simulink library "TM_DynamicModel_Library"  (Simulink 7.8)
settings: Solver=ode45  StartTime=0.0  StopTime=10.0  RelTol=1e-3
undefined symbols (not defined in the file or in its folder): DiscIntNeverNeededParam
libraries: simulink x43, TM_DynamicModel_Library x7
(part 1 of 2)
settings Model: Creator=vpadmaj  LastModifiedBy=vpadmaj

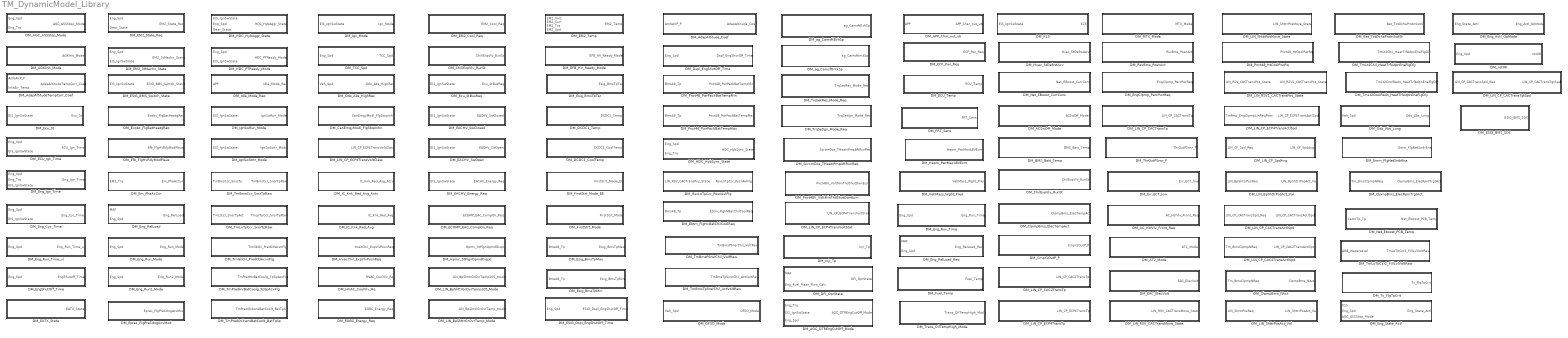
== system TM_DynamicModel_Library ==
  DM_ACSwOff_Mode : Subsystem
  DM_AC_HtrVlv_Front_Req : Subsystem
  DM_AGC_ASSStop_Mode : Subsystem
  DM_AGC_DTREngCutOff_Mode : Subsystem
  DM_AGKInit_Mode : Subsystem
  DM_APP_Char_out_ub : Subsystem
  DM_AT2_Mode : Subsystem
  DM_AdapAltitudeTempCorr_Coef : Subsystem
  DM_AdapAltitude_Coef : Subsystem
  DM_BMS_Batt_Temp : Subsystem
  DM_Bat_TotDchaProtnSwtSt : Subsystem
  DM_CanEmgyModl_FlgStopInhn : Subsystem
  DM_ChilExpVlv_RunSt : Subsystem
  DM_ChillExpVlv_RunSt : Subsystem
  DM_ClpmpBms_ElecRpmTrgtAct : Subsystem
  DM_ClpmpBms_ElecTempAct : Subsystem
  DM_ClpmpBms_NAct : Subsystem
  DM_Cmpr1OutP_P : Subsystem
  DM_DCDC1_CoolTemp : Subsystem
  DM_DCDC1_Temp : Subsystem
  DM_DFI_OprState : Subsystem
  DM_DFSO_Mode : Subsystem
  DM_Dspl_EngShutOff_Time : Subsystem
  DM_EACHV_Energy_Req : Subsystem
  DM_EACHV_SwClosed : Subsystem
  DM_EACHV_SwOpen : Subsystem
  DM_EAC_ElecVolt : Subsystem
  DM_EATX_State : Subsystem
  DM_ECF_Pwr_Req : Subsystem
  DM_ECOMP_EAC_CompOn_Req : Subsystem
  DM_ECU_Ign_Time : Subsystem
  DM_ECU_Temp : Subsystem
  DM_EFB_HV_Ready_Mode : Subsystem
  DM_EM2_Cool_Req : Subsystem
  DM_EM2_StMachn_State : Subsystem
  DM_EM2_State_Req : Subsystem
  DM_EM2_Temp : Subsystem
  DM_EOBC_Energy_Req : Subsystem
  DM_ESIG_BMS_SOC : Subsystem
  DM_ESIG_BMS_Switch_State : Subsystem
  DM_ESIG_Dspl_EngShutOff_Time : Subsystem
  DM_Ebtm_FlgHvBatChilCoolReq : Subsystem
  DM_Ecobc_FlgBatHeatgReq : Subsystem
  DM_Ecu_St : Subsystem
  DM_Ecu_StBusReq : Subsystem
  DM_Efb_FlgHvRdyModPlaus : Subsystem
  DM_Em_PhaAcCur : Subsystem
  DM_Emm_FlgNetSndrEna : Subsystem
  DM_EngClpmp_PercPwrReq : Subsystem
  DM_EngShutOff_Time : Subsystem
  DM_Eng_Actl_OpMode : Subsystem
  DM_Eng_Cyc_Time : Subsystem
  DM_Eng_Ign_Time : Subsystem
  DM_Eng_RelLoad : Subsystem
  DM_Eng_RelLoad_Req : Subsystem
  DM_Eng_Run2_Mode : Subsystem
  DM_Eng_Run_Mode : Subsystem
  DM_Eng_Run_Time : Subsystem
  DM_Eng_Run_Time_ul : Subsystem
  DM_Eng_State_Actl : Subsystem
  DM_Eprec_FlgPreCdngAcvMod : Subsystem
  DM_Err_ECT_low : Subsystem
  DM_Esig_BmsTpMax : Subsystem
  DM_Esig_BmsTpMin : Subsystem
  DM_Esig_BmsTpTar : Subsystem
  DM_FRT_Sens : Subsystem
  DM_FirstStrt_Mode : Subsystem
  DM_FirstStrt_Mode_EE : Subsystem
  DM_Fuel_Temp : Subsystem
  DM_HDC_HybAggr_State : Subsystem
  DM_HDC_HybSync_State : Subsystem
  DM_HDC_PTReady_Mode : Subsystem
  DM_HVAC_CoolVlv_Rq : Subsystem
  DM_Hepm_PwrMax48VEcm : Subsystem
  DM_Hpmc_StPlgnOpmdDispd : Subsystem
  DM_HvacChil_ExpVlvPosnReq : Subsystem
  DM_Hvac_StDefrstAcv : Subsystem
  DM_IC_Knk_Red_Avg : Subsystem
  DM_IC_Knk_Red_Avg_Actv : Subsystem
  DM_Idle_Mode_Req : Subsystem
  DM_IgnSwRun_Mode : Subsystem
  DM_IgnSwStrtr_Mode : Subsystem
  DM_Ign_Mode : Subsystem
  DM_Injr_Tp : Subsystem
  DM_K15 : Subsystem
  DM_LIN_BpShttrGrOvrTemp105_Mode : Subsystem
  DM_LIN_BpShttrGrOvrTemp_Mode : Subsystem
  DM_LIN_BpShttrPosAct_Val : Subsystem
  DM_LIN_CF_SpdAvg : Subsystem
  DM_LIN_CP_CAC2TransActlSpd : Subsystem
  DM_LIN_CP_CAC2TransTp : Subsystem
  DM_LIN_CP_CACTransActlSpd : Subsystem
  DM_LIN_CP_CACTransTgtSpd : Subsystem
  DM_LIN_CP_CACTransTp : Subsystem
  DM_LIN_CP_ECP4TransActlSpd : Subsystem
  DM_LIN_CP_ECP4TransTp : Subsystem
  DM_LIN_CP_ECP4TransVoltClass : Subsystem
  DM_LIN_CP_ECP4TransVoltStat : Subsystem
  DM_LIN_RSV1_CACTransPos_State : Subsystem
  DM_LIN_RSV_CACTransMove_State : Subsystem
  DM_LIN_ShttrPosAct_Val : Subsystem
  DM_LIN_ShttrPosMove_State : Subsystem
  DM_MTX_Mode : Subsystem
  DM_Net_EBoost_CurrCons : Subsystem
  DM_Net_Eboost_PCB_Temp : Subsystem
  DM_Odo_Abs_HighRes : Subsystem
  DM_Odo_Abs_Long : Subsystem
  DM_Pnct48V_VoltMinThdShutDwnEcm : Subsystem
  DM_Pnct48_HtCoolPwrRq : Subsystem
  DM_Pnct48_PwrPackBatTempMax : Subsystem
  DM_Pnct48_PwrPackBatTempMin : Subsystem
  DM_RsvBms_PosnAct : Subsystem
  DM_RsvLoTpCcr_PosnAvlFlg : Subsystem
  DM_ScrcmDos_THeatrPmpAftRunReq : Subsystem
  DM_TCC_Spd : Subsystem
  DM_Tc_FlgTpCrit : Subsystem
  DM_ThrOutPSnsr_P : Subsystem
  DM_TmBmsCcr_SnsrTpRaw : Subsystem
  DM_TmBmsPSnsrChil_VoltRaw : Subsystem
  DM_TmBmsTpSnsrChil_ActVoltRaw : Subsystem
  DM_TmGbOil_PredCtlAcvnFlg : Subsystem
  DM_TmLoTpCcr2_FillLvlVoltRaw : Subsystem
  DM_TmLoTpCcr_SnsrTpRaw : Subsystem
  DM_TmLt2Chil_HeatTrfAdpnEnaFlgDly : Subsystem
  DM_TmLt2CoolRedn_HeatTrfAdpnEnaFlgDly : Subsystem
  DM_TmPredHvBatCoolg_TpSpAcvFlg : Subsystem
  DM_TmPredQckwnsBatCoolt_BatTpSp : Subsystem
  DM_Trans_OilTempHigh_Mode : Subsystem
  DM_TrqSetIgn_Mode_Req : Subsystem
  DM_TrqSetRes_Mode_Req : Subsystem
  DM_VehMass_Wght_Pred : Subsystem
  DM_ag_CamsftExhSp : Subsystem
  DM_ag_CamsftIntkSp : Subsystem
  DM_nst08 : Subsystem

== system TM_DynamicModel_Library/DM_ACSwOff_Mode ==
  Constant : Constant
  ACSwOff_Mode : Outport
  wires:
  Constant/1 -> ACSwOff_Mode/1

== system TM_DynamicModel_Library/DM_AC_HtrVlv_Front_Req ==
  Constant : Constant
  AC_HtrVlv_Front_Req : Outport
  wires:
  Constant/1 -> AC_HtrVlv_Front_Req/1

== system TM_DynamicModel_Library/DM_AGC_ASSStop_Mode ==
  Eng_Spd : Inport
  Eng_Trq : Inport  Port=2
  Add : Sum  Inputs=+-
  Constant : Constant  Value=0
  Constant1 : Constant  Value=-100
  Constant2 : Constant  Value=0
  Data Type Conversion : DataTypeConversion
  Logical Operator : Logic  AllPortsSameDT=off  OutDataTypeStr=boolean
  Logical Operator1 : Logic  Operator=NOR  AllPortsSameDT=off  OutDataTypeStr=boolean
  Relational Operator : RelationalOperator  Operator=>  OutDataTypeStr=boolean
  Relational Operator1 : RelationalOperator  Operator=<  OutDataTypeStr=boolean
  Relational Operator2 : RelationalOperator  Operator=>  OutDataTypeStr=boolean
  Unit Delay : UnitDelay  SampleTime=-1
  AGC_ASSStop_Mode : Outport
  wires:
  Data Type Conversion/1 -> AGC_ASSStop_Mode/1
  Constant/1 -> Relational Operator/2
  Eng_Spd/1 -> Relational Operator/1, Unit Delay/1, Add/1
  Relational Operator/1 -> Logical Operator1/1
  Unit Delay/1 -> Add/2
  Constant1/1 -> Relational Operator1/2
  Add/1 -> Relational Operator1/1
  Constant2/1 -> Relational Operator2/2
  Eng_Trq/1 -> Relational Operator2/1
  Relational Operator1/1 -> Logical Operator/1
  Relational Operator2/1 -> Logical Operator/2
  Logical Operator/1 -> Logical Operator1/2
  Logical Operator1/1 -> Data Type Conversion/1

== system TM_DynamicModel_Library/DM_AGC_DTREngCutOff_Mode ==
  Eng_Trq : Inport
  EIS_IgnSwState : Inport  Port=2
  Eng_Spd : Inport  Port=3
  Constant3 : Constant  Value=0
  DM_AGC_ASSStop_Mode : TM_DynamicModel_Library/DM_AGC_ASSStop_Mode
  DM_Ign_Mode : Subsystem
  Data Type Conversion : DataTypeConversion
  Logical Operator1 : Logic  AllPortsSameDT=off  OutDataTypeStr=boolean
  Logical Operator2 : Logic  Operator=OR  AllPortsSameDT=off  OutDataTypeStr=boolean
  Relational Operator4 : RelationalOperator  Operator=<=  OutDataTypeStr=boolean
  AGC_DTREngCutOff_Mode : Outport
  wires:
  Data Type Conversion/1 -> AGC_DTREngCutOff_Mode/1
  Constant3/1 -> Relational Operator4/2
  Eng_Spd/1 -> Relational Operator4/1, DM_AGC_ASSStop_Mode/1
  Relational Operator4/1 -> Logical Operator1/2
  Logical Operator1/1 -> Logical Operator2/2
  Logical Operator2/1 -> Data Type Conversion/1
  DM_AGC_ASSStop_Mode/1 -> Logical Operator2/1
  EIS_IgnSwState/1 -> DM_Ign_Mode/1(EIS_IgnSwState)
  Eng_Trq/1 -> DM_AGC_ASSStop_Mode/2
  DM_Ign_Mode/1(Ign_Mode) -> Logical Operator1/1

== system TM_DynamicModel_Library/DM_AGKInit_Mode ==
  note: This variable is a part of DC_SP function. Current implementation is from page 1210
      | of function definition document for M256 16A_Star23_VC05 L03FRG
  0 : UnitDelay  SampleTime=-1
  1 : UnitDelay  X0=1  SampleTime=-1
  Add : Sum
  Constant : Constant
  Constant1 : Constant  Value=0
  Data Type Conversion : DataTypeConversion
  Logical Operator : Logic  Operator=NOT  AllPortsSameDT=off  OutDataTypeStr=boolean
  Logical Operator1 : Logic  AllPortsSameDT=off  OutDataTypeStr=boolean
  Relational Operator : RelationalOperator  Operator===  OutDataTypeStr=boolean
  Switch : Switch  Threshold=1
  "This constant value has been changed from 10 to 1, because this function is now being called every 0.1s instead of 0.01s" : Constant  Value=10
  AGKInit_Mode : Outport
  wires:
  Data Type Conversion/1 -> AGKInit_Mode/1
  Switch/1 -> Add/2
  Add/1 -> 0/1
  "This constant value has been changed from 10 to 1, because this function is now being called every 0.1s instead of 0.01s"/1 -> Relational Operator/2
  0/1 -> Relational Operator/1, Add/1
  Relational Operator/1 -> Logical Operator/1, Switch/2
  Logical Operator/1 -> Logical Operator1/1
  1/1 -> Logical Operator1/2
  Logical Operator1/1 -> Data Type Conversion/1, 1/1
  Constant1/1 -> Switch/1
  Constant/1 -> Switch/3

== system TM_DynamicModel_Library/DM_APP_Char_out_ub ==
  APP : Inport
  Characterisation : Lookup  InputValues=[0,10,20,30,40,50,60,70,80,90,100]  Table=[0,8,17,26,35,44,59,70,82,91,100]
  APP_Char_out_ub : Outport
  wires:
  APP/1 -> Characterisation/1
  Characterisation/1 -> APP_Char_out_ub/1

== system TM_DynamicModel_Library/DM_AT2_Mode ==
  Constant : Constant  Value=0
  AT2_Mode : Outport
  wires:
  Constant/1 -> AT2_Mode/1

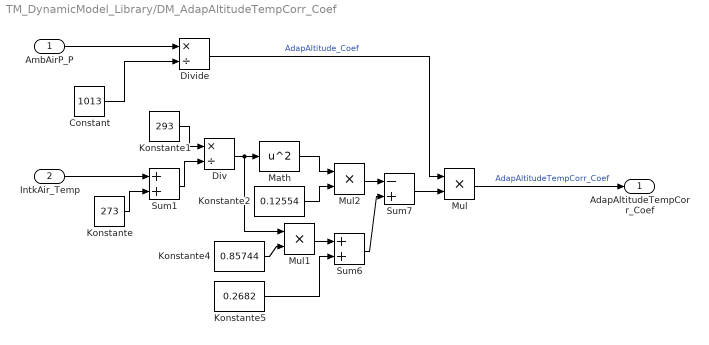
== system TM_DynamicModel_Library/DM_AdapAltitudeTempCorr_Coef ==
  AmbAirP_P : Inport
  IntkAir_Temp : Inport  Port=2  PortDimensions=1
  Constant : Constant  Value=1013
  Div : Product  Tag=COPIED_DURING_UPGRADE  Description=|  Inputs=*/  RndMeth=Zero  mask(TL_Product){data={'logdata',{'plotchannels',[]},'output',{'type','DC_FCTR_32768_U16'},'date',734244.44671856484}}
      | Product block of dSPACE TargetLink.
      | 
      | Output signal is equal to the product of the input signals. The input ports are specified according to conventions for Simulink Product blocks.
      settings: DeleteFcn=if exist('delete_tlblock','file')==2,delete_tlblock(gcbh);end  NameChangeFcn=if exist('rename_tlblock','file')==2,rename_tlblock(gcbh);end  OpenFcn=if exist('tl_open_blockdlg','file')==2,tl_open_blockdlg(gcbh);else,open_system(gcbh,'parameter');end
      mask Help: eval(['if exist(''tl_online_help'',''file'') == 2, tl_online_help(''Topic'',''TL_Product''),else, web([''jar:file:///'',matlabroot,''/help/toolbox/simulink/help.jar!/slref/' lower(get_param(gcbh,'Blocktype')) '.html''], ''-helpbrowser''),end'])
  Divide : Product  Inputs=*/
  Konstante : Constant  Tag=COPIED_DURING_UPGRADE  Description=|  Value=273
      | Constant block of dSPACE TargetLink.
      | 
      | Output signal keeps the given constant value.
      settings: DeleteFcn=if exist('delete_tlblock','file')==2,delete_tlblock(gcbh);end  NameChangeFcn=if exist('rename_tlblock','file')==2,rename_tlblock(gcbh);end  OpenFcn=if exist('tl_open_blockdlg','file')==2,tl_open_blockdlg(gcbh);else,open_system(gcbh,'parameter');end
  Konstante1 : Constant  Tag=COPIED_DURING_UPGRADE  Description=|  Value=293  mask(TL_Constant){data={'date',734244.44671675924}}
      | Constant block of dSPACE TargetLink.
      | 
      | Output signal keeps the given constant value.
      settings: DeleteFcn=if exist('delete_tlblock','file')==2,delete_tlblock(gcbh);end  NameChangeFcn=if exist('rename_tlblock','file')==2,rename_tlblock(gcbh);end  OpenFcn=if exist('tl_open_blockdlg','file')==2,tl_open_blockdlg(gcbh);else,open_system(gcbh,'parameter');end
      mask Help: eval(['if exist(''tl_online_help'',''file'') == 2, tl_online_help(''Topic'',''TL_Constant''),else, web([''jar:file:///'',matlabroot,''/help/toolbox/simulink/help.jar!/slref/' lower(get_param(gcbh,'Blocktype')) '.html''], ''-helpbrowser''),end'])
  Konstante2 : Constant  Tag=COPIED_DURING_UPGRADE  Description=|  Value=0.12554
      | Constant block of dSPACE TargetLink.
      | 
      | Output signal keeps the given constant value.
      settings: DeleteFcn=if exist('delete_tlblock','file')==2,delete_tlblock(gcbh);end  NameChangeFcn=if exist('rename_tlblock','file')==2,rename_tlblock(gcbh);end  OpenFcn=if exist('tl_open_blockdlg','file')==2,tl_open_blockdlg(gcbh);else,open_system(gcbh,'parameter');end
  Konstante4 : Constant  Tag=COPIED_DURING_UPGRADE  Description=|  Value=0.85744
      | Constant block of dSPACE TargetLink.
      | 
      | Output signal keeps the given constant value.
      settings: DeleteFcn=if exist('delete_tlblock','file')==2,delete_tlblock(gcbh);end  NameChangeFcn=if exist('rename_tlblock','file')==2,rename_tlblock(gcbh);end  OpenFcn=if exist('tl_open_blockdlg','file')==2,tl_open_blockdlg(gcbh);else,open_system(gcbh,'parameter');end
  Konstante5 : Constant  Tag=COPIED_DURING_UPGRADE  Description=|  Value=0.2682
      | Constant block of dSPACE TargetLink.
      | 
      | Output signal keeps the given constant value.
      settings: DeleteFcn=if exist('delete_tlblock','file')==2,delete_tlblock(gcbh);end  NameChangeFcn=if exist('rename_tlblock','file')==2,rename_tlblock(gcbh);end  OpenFcn=if exist('tl_open_blockdlg','file')==2,tl_open_blockdlg(gcbh);else,open_system(gcbh,'parameter');end
  Math : Math  Tag=COPIED_DURING_UPGRADE  Description=|  Operator=square  SaturateOnIntegerOverflow=on
      | Math block of dSPACE TargetLink.
      | 
      | The Math block outputs the result of the specified math function applied to the input(s). Note that unlike Simulink's Math block, this block does not support complex signals.
      settings: DeleteFcn=if exist('delete_tlblock','file')==2,delete_tlblock(gcbh);end  NameChangeFcn=if exist('rename_tlblock','file')==2,rename_tlblock(gcbh);end  OpenFcn=if exist('tl_open_blockdlg','file')==2,tl_open_blockdlg(gcbh);else,open_system(gcbh,'parameter');end
  Mul : Product  Tag=COPIED_DURING_UPGRADE  Description=|  RndMeth=Zero
      | Product block of dSPACE TargetLink.
      | 
      | Output signal is equal to the product of the input signals. The input ports are specified according to conventions for Simulink Product blocks.
      settings: DeleteFcn=if exist('delete_tlblock','file')==2,delete_tlblock(gcbh);end  NameChangeFcn=if exist('rename_tlblock','file')==2,rename_tlblock(gcbh);end  OpenFcn=if exist('tl_open_blockdlg','file')==2,tl_open_blockdlg(gcbh);else,open_system(gcbh,'parameter');end
  Mul1 : Product  Tag=COPIED_DURING_UPGRADE  Description=|  RndMeth=Zero
      | Product block of dSPACE TargetLink.
      | 
      | Output signal is equal to the product of the input signals. The input ports are specified according to conventions for Simulink Product blocks.
      settings: DeleteFcn=if exist('delete_tlblock','file')==2,delete_tlblock(gcbh);end  NameChangeFcn=if exist('rename_tlblock','file')==2,rename_tlblock(gcbh);end  OpenFcn=if exist('tl_open_blockdlg','file')==2,tl_open_blockdlg(gcbh);else,open_system(gcbh,'parameter');end
  Mul2 : Product  Tag=COPIED_DURING_UPGRADE  Description=|  RndMeth=Zero
      | Product block of dSPACE TargetLink.
      | 
      | Output signal is equal to the product of the input signals. The input ports are specified according to conventions for Simulink Product blocks.
      settings: DeleteFcn=if exist('delete_tlblock','file')==2,delete_tlblock(gcbh);end  NameChangeFcn=if exist('rename_tlblock','file')==2,rename_tlblock(gcbh);end  OpenFcn=if exist('tl_open_blockdlg','file')==2,tl_open_blockdlg(gcbh);else,open_system(gcbh,'parameter');end
  Sum1 : Sum  Tag=COPIED_DURING_UPGRADE  Description=|
      | Sum block of dSPACE TargetLink.
      | 
      | Output signal is equal to the sum of the input signals.
      | The list of signs is specified according to conventions for Simulink Sum blocks.
      settings: DeleteFcn=if exist('delete_tlblock','file')==2,delete_tlblock(gcbh);end  NameChangeFcn=if exist('rename_tlblock','file')==2,rename_tlblock(gcbh);end  OpenFcn=if exist('tl_open_blockdlg','file')==2,tl_open_blockdlg(gcbh);else,open_system(gcbh,'parameter');end
  Sum6 : Sum  Tag=COPIED_DURING_UPGRADE  Description=|
      | Sum block of dSPACE TargetLink.
      | 
      | Output signal is equal to the sum of the input signals.
      | The list of signs is specified according to conventions for Simulink Sum blocks.
      settings: DeleteFcn=if exist('delete_tlblock','file')==2,delete_tlblock(gcbh);end  NameChangeFcn=if exist('rename_tlblock','file')==2,rename_tlblock(gcbh);end  OpenFcn=if exist('tl_open_blockdlg','file')==2,tl_open_blockdlg(gcbh);else,open_system(gcbh,'parameter');end
  Sum7 : Sum  Tag=COPIED_DURING_UPGRADE  Description=|  Inputs=-+
      | Sum block of dSPACE TargetLink.
      | 
      | Output signal is equal to the sum of the input signals.
      | The list of signs is specified according to conventions for Simulink Sum blocks.
      settings: DeleteFcn=if exist('delete_tlblock','file')==2,delete_tlblock(gcbh);end  NameChangeFcn=if exist('rename_tlblock','file')==2,rename_tlblock(gcbh);end  OpenFcn=if exist('tl_open_blockdlg','file')==2,tl_open_blockdlg(gcbh);else,open_system(gcbh,'parameter');end
  AdapAltitudeTempCorr_Coef : Outport
  wires:
  AmbAirP_P/1 -> Divide/1
  IntkAir_Temp/1 -> Sum1/1
  Mul/1 -> AdapAltitudeTempCorr_Coef/1  "AdapAltitudeTempCorr_Coef"
  Constant/1 -> Divide/2
  Sum7/1 -> Mul/2
  Mul2/1 -> Sum7/1
  Sum6/1 -> Sum7/2
  Math/1 -> Mul2/1
  Div/1 -> Mul1/1, Math/1
  Konstante2/1 -> Mul2/2
  Konstante4/1 -> Mul1/2
  Mul1/1 -> Sum6/1
  Konstante5/1 -> Sum6/2
  Konstante1/1 -> Div/1
  Sum1/1 -> Div/2
  Konstante/1 -> Sum1/2
  Divide/1 -> Mul/1  "AdapAltitude_Coef"

== system TM_DynamicModel_Library/DM_AdapAltitude_Coef ==
  AmbAirP_P : Inport
  Constant : Constant  Value=1013
  Divide : Product  Inputs=*/
  AdapAltitude_Coef : Outport
  wires:
  AmbAirP_P/1 -> Divide/1
  Constant/1 -> Divide/2
  Divide/1 -> AdapAltitude_Coef/1  "AdapAltitude_Coef"

== system TM_DynamicModel_Library/DM_BMS_Batt_Temp ==
  Constant : Constant  Value=30
  BMS_Batt_Temp : Outport
  wires:
  Constant/1 -> BMS_Batt_Temp/1

== system TM_DynamicModel_Library/DM_Bat_TotDchaProtnSwtSt ==
  Constant : Constant
  Bat_TotDchaProtnSwtSt : Outport
  wires:
  Constant/1 -> Bat_TotDchaProtnSwtSt/1

== system TM_DynamicModel_Library/DM_CanEmgyModl_FlgStopInhn ==
  Constant : Constant  Value=0
  CanEmgyModl_FlgStopInhn : Outport
  wires:
  Constant/1 -> CanEmgyModl_FlgStopInhn/1

== system TM_DynamicModel_Library/DM_ChilExpVlv_RunSt ==
  Constant : Constant  Value=0
  ChilExpVlv_RunSt : Outport
  wires:
  Constant/1 -> ChilExpVlv_RunSt/1

== system TM_DynamicModel_Library/DM_ChillExpVlv_RunSt ==
  Constant : Constant  Value=0
  ChillExpVlv_RunSt : Outport
  wires:
  Constant/1 -> ChillExpVlv_RunSt/1

== system TM_DynamicModel_Library/DM_ClpmpBms_ElecRpmTrgtAct ==
  Tm_BmsClpmpNReq : Inport
  Unit Delay : UnitDelay  SampleTime=-1
  ClpmpBms_ElecRpmTrgtAct : Outport
  wires:
  Unit Delay/1 -> ClpmpBms_ElecRpmTrgtAct/1
  Tm_BmsClpmpNReq/1 -> Unit Delay/1

== system TM_DynamicModel_Library/DM_ClpmpBms_ElecTempAct ==
  Constant : Constant  Value=40
  ClpmpBms_ElecTempAct : Outport
  wires:
  Constant/1 -> ClpmpBms_ElecTempAct/1

== system TM_DynamicModel_Library/DM_ClpmpBms_NAct ==
  Tm_BmsClpmpNReq : Inport
  Unit Delay : UnitDelay  SampleTime=-1
  Unit Delay1 : UnitDelay  SampleTime=-1
  ClpmpBms_NAct : Outport
  wires:
  Tm_BmsClpmpNReq/1 -> Unit Delay/1
  Unit Delay/1 -> Unit Delay1/1
  Unit Delay1/1 -> ClpmpBms_NAct/1

== system TM_DynamicModel_Library/DM_Cmpr1OutP_P ==
  Constant : Constant  Value=1000
  Cmpr1OutP_P : Outport
  wires:
  Constant/1 -> Cmpr1OutP_P/1

== system TM_DynamicModel_Library/DM_DCDC1_CoolTemp ==
  Constant : Constant  Value=30
  DCDC1_CoolTemp : Outport
  wires:
  Constant/1 -> DCDC1_CoolTemp/1

== system TM_DynamicModel_Library/DM_DCDC1_Temp ==
  Constant : Constant  Value=30
  DCDC1_Temp : Outport
  wires:
  Constant/1 -> DCDC1_Temp/1

== system TM_DynamicModel_Library/DM_DFI_OprState ==
  MAF : Inport
  Eng_Fuel_Mass_Flow_Calc : Inport  Port=2
  Constant : Constant  Value=65
  Constant1 : Constant
  Constant2 : Constant  Value=1.06
  Divide : Product  Inputs=*/
  Relational Operator : RelationalOperator  Operator=<  OutDataTypeStr=boolean
  Saturation : Saturate  UpperLimit=inf  LowerLimit=eps
  Switch : Switch
  kgph_2_gpmin : Gain  Gain=60/1000
  DFI_OprState : Outport
  wires:
  kgph_2_gpmin/1 -> Divide/1
  MAF/1 -> kgph_2_gpmin/1
  Eng_Fuel_Mass_Flow_Calc/1 -> Saturation/1
  Divide/1 -> Relational Operator/1
  Relational Operator/1 -> Switch/2
  Switch/1 -> DFI_OprState/1
  Constant/1 -> Switch/1
  Constant1/1 -> Switch/3
  Constant2/1 -> Relational Operator/2
  Saturation/1 -> Divide/2

== system TM_DynamicModel_Library/DM_DFSO_Mode ==
  Veh_Spd : Inport
  Constant1 : Constant  Value=-0.7
  Data Type Conversion : DataTypeConversion
  Derivative : Derivative
  Gain2 : Gain  Gain=0.4
  Relational Operator : RelationalOperator  OutDataTypeStr=boolean
  DFSO_Mode : Outport
  wires:
  Data Type Conversion/1 -> DFSO_Mode/1
  Derivative/1 -> Gain2/1
  Gain2/1 -> Relational Operator/2
  Constant1/1 -> Relational Operator/1
  Relational Operator/1 -> Data Type Conversion/1
  Veh_Spd/1 -> Derivative/1

== system TM_DynamicModel_Library/DM_Dspl_EngShutOff_Time ==
  Eng_Spd : Inport
  DM_EngShutoff_Time : Subsystem
  Dspl_EngShutOff_Time : Outport
  wires:
  Eng_Spd/1 -> DM_EngShutoff_Time/1(Eng_Spd)
  DM_EngShutoff_Time/1(EngShutoff_Time) -> Dspl_EngShutOff_Time/1

== system TM_DynamicModel_Library/DM_EACHV_Energy_Req ==
  EIS_IgnSwState : Inport
  Constant : Constant  Value=4
  DM_Ecu_St : Subsystem
  Data Type Conversion : DataTypeConversion
  Relational Operator : RelationalOperator  Operator===  OutDataTypeStr=boolean
  EACHV_Energy_Req : Outport
  wires:
  Data Type Conversion/1 -> EACHV_Energy_Req/1
  Constant/1 -> Relational Operator/2
  Relational Operator/1 -> Data Type Conversion/1
  EIS_IgnSwState/1 -> DM_Ecu_St/1(EIS_IgnSwState)
  DM_Ecu_St/1(Ecu_St) -> Relational Operator/1

== system TM_DynamicModel_Library/DM_EACHV_SwClosed ==
  EIS_IgnSwState : Inport
  Constant : Constant  Value=2
  DM_ESIG_BMS_Switch_State : Subsystem
  Data Type Conversion : DataTypeConversion
  Relational Operator : RelationalOperator  Operator===  OutDataTypeStr=boolean
  EACHV_SwClosed : Outport
  wires:
  Data Type Conversion/1 -> EACHV_SwClosed/1
  Constant/1 -> Relational Operator/2
  Relational Operator/1 -> Data Type Conversion/1
  EIS_IgnSwState/1 -> DM_ESIG_BMS_Switch_State/1(EIS_IgnSwState)
  DM_ESIG_BMS_Switch_State/1(ESIG_BMS_Switch_State) -> Relational Operator/1

== system TM_DynamicModel_Library/DM_EACHV_SwOpen ==
  EIS_IgnSwState : Inport
  Constant : Constant  Value=2
  DM_ESIG_BMS_Switch_State : Subsystem
  Data Type Conversion : DataTypeConversion
  Logical Operator : Logic  Operator=NOT  AllPortsSameDT=off  OutDataTypeStr=boolean
  Relational Operator : RelationalOperator  Operator===  OutDataTypeStr=boolean
  EACHV_SwOpen : Outport
  wires:
  Data Type Conversion/1 -> EACHV_SwOpen/1
  Constant/1 -> Relational Operator/2
  Relational Operator/1 -> Logical Operator/1
  Logical Operator/1 -> Data Type Conversion/1
  EIS_IgnSwState/1 -> DM_ESIG_BMS_Switch_State/1(EIS_IgnSwState)
  DM_ESIG_BMS_Switch_State/1(ESIG_BMS_Switch_State) -> Relational Operator/1

== system TM_DynamicModel_Library/DM_EAC_ElecVolt ==
  Constant : Constant  Value=48
  EAC_ElecVolt : Outport
  wires:
  Constant/1 -> EAC_ElecVolt/1

== system TM_DynamicModel_Library/DM_EATX_State ==
  Constant : Constant  Value=4
  EATX_State : Outport
  wires:
  Constant/1 -> EATX_State/1

== system TM_DynamicModel_Library/DM_ECF_Pwr_Req ==
  Constant : Constant  Value=0
  ECF_Pwr_Req : Outport
  wires:
  Constant/1 -> ECF_Pwr_Req/1

== system TM_DynamicModel_Library/DM_ECOMP_EAC_CompOn_Req ==
  Constant : Constant  Value=0
  ECOMP_EAC_CompOn_Req : Outport
  wires:
  Constant/1 -> ECOMP_EAC_CompOn_Req/1

== system TM_DynamicModel_Library/DM_ECU_Ign_Time ==
  Eng_Spd : Inport
  EIS_IgnSwState : Inport  Port=2
  Constant46 : Constant  Value=0
  Constant47 : Constant  Value=0
  Constant48 : Constant  Value=0
  Counter_RE : Subsystem
  EdgeBi : Subsystem
  Eng_Run2_Mode_Sys : TM_DynamicModel_Library/DM_Eng_Run2_Mode
  Gain : Gain  Gain=0.01
  IgnSwRun_Mode : Subsystem
  Unit Delay3 : UnitDelay  SampleTime=-1
  ECU_Ign_Time : Outport
  wires:
  Constant46/1 -> Counter_RE/3(InitVal)
  EdgeBi/1(y) -> Counter_RE/2(Reset)
  Unit Delay3/1 -> EdgeBi/2(R)
  Constant47/1 -> EdgeBi/3(IV)
  Constant48/1 -> Unit Delay3/1
  Eng_Run2_Mode_Sys/1 -> Counter_RE/1(Enable)
  Counter_RE/1(y) -> Gain/1
  Gain/1 -> ECU_Ign_Time/1
  Eng_Spd/1 -> Eng_Run2_Mode_Sys/1
  IgnSwRun_Mode/1(IgnSwRun_Mode) -> EdgeBi/1(u)
  EIS_IgnSwState/1 -> IgnSwRun_Mode/1(IgnKeyPosition)

== system TM_DynamicModel_Library/DM_ECU_Temp ==
  Constant : Constant  Value=30
  ECU_Temp : Outport
  wires:
  Constant/1 -> ECU_Temp/1

== system TM_DynamicModel_Library/DM_EFB_HV_Ready_Mode ==
  Constant : Constant
  EFB_HV_Ready_Mode : Outport
  wires:
  Constant/1 -> EFB_HV_Ready_Mode/1

== system TM_DynamicModel_Library/DM_EM2_Cool_Req ==
  Constant : Constant  Value=0
  EM2_Cool_Req : Outport
  wires:
  Constant/1 -> EM2_Cool_Req/1

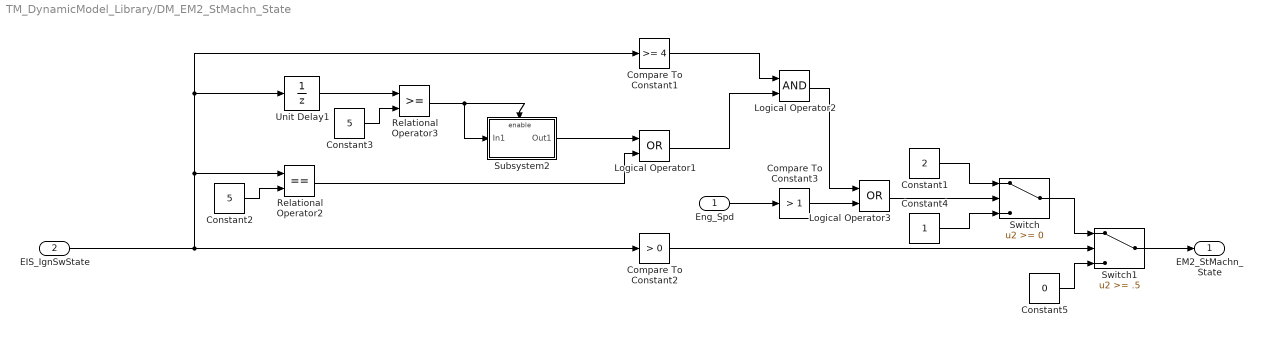
== system TM_DynamicModel_Library/DM_EM2_StMachn_State ==
  Eng_Spd : Inport
  EIS_IgnSwState : Inport  Port=2
  Compare To Constant1 : simulink/Logic and Bit Operations/Compare To Constant  relop=>=  const=4  OutDataTypeStr=uint8
  Compare To Constant2 : simulink/Logic and Bit Operations/Compare To Constant  relop=>  const=0  OutDataTypeStr=uint8
  Compare To Constant3 : simulink/Logic and Bit Operations/Compare To Constant  relop=>  const=1  OutDataTypeStr=uint8
  Constant1 : Constant  Value=2
  Constant2 : Constant  Value=5
  Constant3 : Constant  Value=5
  Constant4 : Constant
  Constant5 : Constant  Value=0
  Logical Operator1 : Logic  Operator=OR  AllPortsSameDT=off  OutDataTypeStr=boolean
  Logical Operator2 : Logic  AllPortsSameDT=off  OutDataTypeStr=boolean
  Logical Operator3 : Logic  Operator=OR  AllPortsSameDT=off  OutDataTypeStr=boolean
  Relational Operator2 : RelationalOperator  Operator===  OutDataTypeStr=boolean
  Relational Operator3 : RelationalOperator  OutDataTypeStr=boolean
  Subsystem2 : Subsystem
  Switch : Switch
  Switch1 : Switch  Threshold=.5
  Unit Delay1 : UnitDelay  SampleTime=-1
  EM2_StMachn_State : Outport
  wires:
  EIS_IgnSwState/1 -> Relational Operator2/1, Compare To Constant1/1, Unit Delay1/1, Compare To Constant2/1
  Constant2/1 -> Relational Operator2/2
  Unit Delay1/1 -> Relational Operator3/1
  Constant3/1 -> Relational Operator3/2
  Relational Operator2/1 -> Logical Operator1/2
  Subsystem2/1(Out1) -> Logical Operator1/1
  Compare To Constant1/1 -> Logical Operator2/1
  Logical Operator1/1 -> Logical Operator2/2
  Constant1/1 -> Switch/1
  Constant4/1 -> Switch/3
  Switch/1 -> Switch1/1
  Constant5/1 -> Switch1/3
  Compare To Constant2/1 -> Switch1/2
  Logical Operator2/1 -> Logical Operator3/1
  Switch1/1 -> EM2_StMachn_State/1
  Relational Operator3/1 -> Subsystem2/1(In1), Subsystem2/Enable
  Logical Operator3/1 -> Switch/2
  Eng_Spd/1 -> Compare To Constant3/1
  Compare To Constant3/1 -> Logical Operator3/2

== system TM_DynamicModel_Library/DM_EM2_State_Req ==
  Eng_Spd : Inport
  Gear_State : Inport  Port=2
  Compare To Constant2 : simulink/Logic and Bit Operations/Compare To Constant  relop=<  const=.1  OutDataTypeStr=uint8
  Compare To Constant3 : simulink/Logic and Bit Operations/Compare To Constant  relop=<  const=.1  OutDataTypeStr=uint8
  Compare To Constant5 : simulink/Logic and Bit Operations/Compare To Constant  relop=>  const=600  OutDataTypeStr=uint8
  Compare To Constant6 : simulink/Logic and Bit Operations/Compare To Constant  relop=>  const=.1  OutDataTypeStr=uint8
  Constant1 : Constant
  Constant6 : Constant
  Constant7 : Constant  Value=6
  Logical Operator1 : Logic  AllPortsSameDT=off  OutDataTypeStr=boolean
  Logical Operator4 : Logic  AllPortsSameDT=off  OutDataTypeStr=boolean
  Switch1 : Switch  Threshold=.5
  Switch2 : Switch  Threshold=.5
  EM2_State_Req : Outport
  wires:
  Gear_State/1 -> Compare To Constant6/1, Compare To Constant3/1
  Eng_Spd/1 -> Compare To Constant2/1, Compare To Constant5/1
  Constant6/1 -> Switch2/1
  Constant7/1 -> Switch2/3
  Compare To Constant3/1 -> Logical Operator1/1
  Compare To Constant2/1 -> Logical Operator1/2
  Logical Operator1/1 -> Switch1/2
  Constant1/1 -> Switch1/1
  Switch2/1 -> Switch1/3
  Compare To Constant5/1 -> Logical Operator4/1
  Compare To Constant6/1 -> Logical Operator4/2
  Logical Operator4/1 -> Switch2/2
  Switch1/1 -> EM2_State_Req/1

== system TM_DynamicModel_Library/DM_EM2_Temp ==
  note: Init Value: 22 - UDDS
      |    63 -  NUR
  EM2_Volt : Inport
  EM2_Curr : Inport  Port=2
  EM2_Trq : Inport  Port=3
  EM2_Spd : Inport  Port=4
  Constant1 : Constant  Value=63
  Discrete-Time Integrator : DiscreteIntegrator  InitialConditionSource=external  InitialCondition=22  SampleTime=0.1  ICPrevOutput=DiscIntNeverNeededParam  ICPrevScaledInput=DiscIntNeverNeededParam
  Gain : Gain  Gain=pi/30
  Gain1 : Gain  Gain=1/(100*1000)
  GainUsedInHIL : Gain  Gain=1/(2*358)
  Ground : Ground
  Subsystem : Subsystem
  Terminator : Terminator
  EM2_Temp : Outport
  wires:
  EM2_Spd/1 -> Gain/1
  EM2_Volt/1 -> Subsystem/1(V)
  EM2_Curr/1 -> Subsystem/2(I)
  EM2_Trq/1 -> Subsystem/3(Trq)
  Subsystem/1(dQ) -> Gain1/1
  Discrete-Time Integrator/1 -> EM2_Temp/1
  Constant1/1 -> Discrete-Time Integrator/2
  Gain1/1 -> Discrete-Time Integrator/1
  Gain/1 -> Subsystem/4(Spd)
  Ground/1 -> GainUsedInHIL/1
  GainUsedInHIL/1 -> Terminator/1

== system TM_DynamicModel_Library/DM_EOBC_Energy_Req ==
  Constant : Constant  Value=0
  EOBC_Energy_Req : Outport
  wires:
  Constant/1 -> EOBC_Energy_Req/1

== system TM_DynamicModel_Library/DM_ESIG_BMS_SOC ==
  Constant : Constant  Value=70
  ESIG_BMS_SOC : Outport
  wires:
  Constant/1 -> ESIG_BMS_SOC/1

== system TM_DynamicModel_Library/DM_ESIG_BMS_Switch_State ==
  EIS_IgnSwState : Inport
  Compare To Constant : simulink/Logic and Bit Operations/Compare To Constant  relop=<  const=1.0  OutDataTypeStr=uint8
  Data Type Conversion : DataTypeConversion
  Delay : Delay  DelayLength=15000  InitialCondition=2  SampleTime=0.1
  Gain : Gain  Gain=2
  Logical Operator : Logic  Operator=NOT  AllPortsSameDT=off  OutDataTypeStr=boolean
  ESIG_BMS_Switch_State : Outport
  wires:
  Data Type Conversion/1 -> ESIG_BMS_Switch_State/1
  EIS_IgnSwState/1 -> Compare To Constant/1
  Delay/1 -> Data Type Conversion/1
  Compare To Constant/1 -> Logical Operator/1
  Logical Operator/1 -> Gain/1
  Gain/1 -> Delay/1

== system TM_DynamicModel_Library/DM_ESIG_Dspl_EngShutOff_Time ==
  Eng_Spd : Inport
  DM_EngShutoff_Time : Subsystem
  ESIG_Dspl_EngShutOff_Time : Outport
  wires:
  DM_EngShutoff_Time/1(EngShutoff_Time) -> ESIG_Dspl_EngShutOff_Time/1
  Eng_Spd/1 -> DM_EngShutoff_Time/1(Eng_Spd)

== system TM_DynamicModel_Library/DM_Ebtm_FlgHvBatChilCoolReq ==
  Bms48_Tp : Inport
  Constant : Constant  Value=36
  Data Type Conversion : DataTypeConversion
  Relational Operator : RelationalOperator  Operator=>  OutDataTypeStr=boolean
  Ebtm_FlgHvBatChilCoolReq : Outport
  wires:
  Data Type Conversion/1 -> Ebtm_FlgHvBatChilCoolReq/1
  Bms48_Tp/1 -> Relational Operator/1
  Constant/1 -> Relational Operator/2
  Relational Operator/1 -> Data Type Conversion/1

== system TM_DynamicModel_Library/DM_Ecobc_FlgBatHeatgReq ==
  Constant : Constant  Value=0
  Ecobc_FlgBatHeatgReq : Outport
  wires:
  Constant/1 -> Ecobc_FlgBatHeatgReq/1

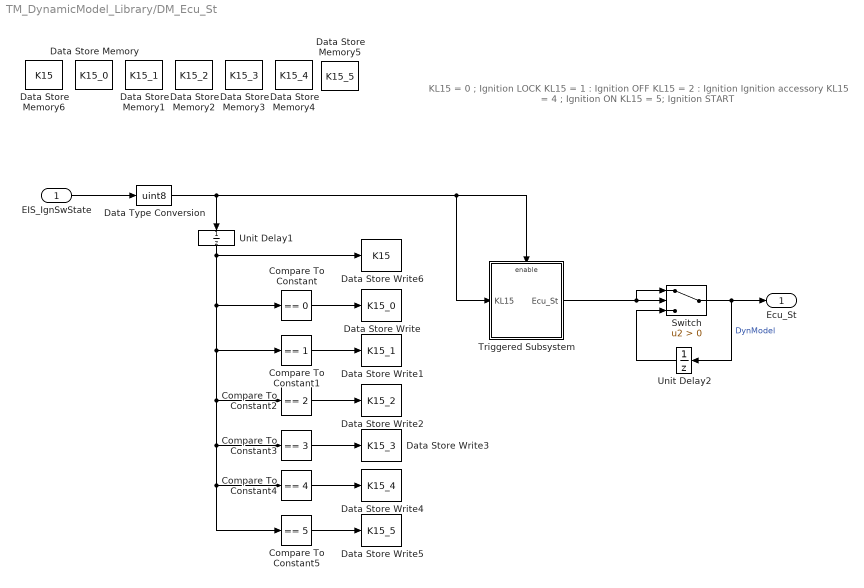
== system TM_DynamicModel_Library/DM_Ecu_St ==
  note: KL15 = 0 ; Ignition LOCK
      | KL15 = 1 : Ignition OFF
      | KL15 = 2 : Ignition Ignition accessory
      | KL15 = 4 ; Ignition ON
      | KL15 = 5; Ignition START
  EIS_IgnSwState : Inport  SampleTime=0.1
  Compare To Constant : simulink/Logic and Bit Operations/Compare To Constant  relop===  const=0  OutDataTypeStr=uint8
  Compare To Constant1 : simulink/Logic and Bit Operations/Compare To Constant  relop===  const=1  OutDataTypeStr=uint8
  Compare To Constant2 : simulink/Logic and Bit Operations/Compare To Constant  relop===  const=2  OutDataTypeStr=uint8
  Compare To Constant3 : simulink/Logic and Bit Operations/Compare To Constant  relop===  const=3  OutDataTypeStr=uint8
  Compare To Constant4 : simulink/Logic and Bit Operations/Compare To Constant  relop===  const=4  OutDataTypeStr=uint8
  Compare To Constant5 : simulink/Logic and Bit Operations/Compare To Constant  relop===  const=5  OutDataTypeStr=uint8
  Data Store Memory : DataStoreMemory  DataStoreName=K15_0  ReadBeforeWriteMsg=warning  WriteAfterWriteMsg=warning  WriteAfterReadMsg=warning
  Data Store Memory1 : DataStoreMemory  DataStoreName=K15_1  ReadBeforeWriteMsg=warning  WriteAfterWriteMsg=warning  WriteAfterReadMsg=warning
  Data Store Memory2 : DataStoreMemory  DataStoreName=K15_2  ReadBeforeWriteMsg=warning  WriteAfterWriteMsg=warning  WriteAfterReadMsg=warning
  Data Store Memory3 : DataStoreMemory  DataStoreName=K15_3  ReadBeforeWriteMsg=warning  WriteAfterWriteMsg=warning  WriteAfterReadMsg=warning
  Data Store Memory4 : DataStoreMemory  DataStoreName=K15_4  ReadBeforeWriteMsg=warning  WriteAfterWriteMsg=warning  WriteAfterReadMsg=warning
  Data Store Memory5 : DataStoreMemory  DataStoreName=K15_5  ReadBeforeWriteMsg=warning  WriteAfterWriteMsg=warning  WriteAfterReadMsg=warning
  Data Store Memory6 : DataStoreMemory  DataStoreName=K15  ReadBeforeWriteMsg=warning  WriteAfterWriteMsg=warning  WriteAfterReadMsg=warning
  Data Store Write : DataStoreWrite  DataStoreName=K15_0
  Data Store Write1 : DataStoreWrite  DataStoreName=K15_1
  Data Store Write2 : DataStoreWrite  DataStoreName=K15_2
  Data Store Write3 : DataStoreWrite  DataStoreName=K15_3
  Data Store Write4 : DataStoreWrite  DataStoreName=K15_4
  Data Store Write5 : DataStoreWrite  DataStoreName=K15_5
  Data Store Write6 : DataStoreWrite  DataStoreName=K15
  Data Type Conversion : DataTypeConversion  OutDataTypeStr=uint8
  Switch : Switch  Criteria=u2 > Threshold
  Triggered Subsystem : Subsystem  TreatAsAtomicUnit=on
  Unit Delay1 : UnitDelay  SampleTime=-1
  Unit Delay2 : UnitDelay  SampleTime=-1
  Ecu_St : Outport  SampleTime=0.1
  wires:
  Data Type Conversion/1 -> Unit Delay1/1, Triggered Subsystem/Enable, Triggered Subsystem/1(KL15)
  Unit Delay1/1 -> Data Store Write6/1, Compare To Constant4/1, Compare To Constant5/1, Compare To Constant3/1, Compare To Constant2/1, Compare To Constant1/1, Compare To Constant/1
  Compare To Constant/1 -> Data Store Write/1
  Compare To Constant1/1 -> Data Store Write1/1
  EIS_IgnSwState/1 -> Data Type Conversion/1
  Compare To Constant2/1 -> Data Store Write2/1
  Compare To Constant3/1 -> Data Store Write3/1
  Compare To Constant4/1 -> Data Store Write4/1
  Compare To Constant5/1 -> Data Store Write5/1
  Triggered Subsystem/1(Ecu_St) -> Switch/2, Switch/1
  Switch/1 -> Unit Delay2/1, Ecu_St/1  "DynModel"
  Unit Delay2/1 -> Switch/3

== system TM_DynamicModel_Library/DM_Ecu_StBusReq ==
  EIS_IgnSwState : Inport
  Constant1 : Constant
  Constant2 : Constant  Value=2
  DM_Ign_Mode : Subsystem
  Switch : Switch  Criteria=u2 > Threshold
  Ecu_StBusReq : Outport
  wires:
  Switch/1 -> Ecu_StBusReq/1
  Constant1/1 -> Switch/1
  Constant2/1 -> Switch/3
  EIS_IgnSwState/1 -> DM_Ign_Mode/1(EIS_IgnSwState)
  DM_Ign_Mode/1(Ign_Mode) -> Switch/2

== system TM_DynamicModel_Library/DM_Efb_FlgHvRdyModPlaus ==
  Constant : Constant  Value=0
  Efb_FlgHvRdyModPlaus : Outport
  wires:
  Constant/1 -> Efb_FlgHvRdyModPlaus/1

== system TM_DynamicModel_Library/DM_Em_PhaAcCur ==
  EM2_Trq : Inport
  1-D Lookup Table : Lookup_n-D  NumberOfTableDimensions=1  BreakpointsForDimension1=[-247 0 231]  Table=[-150 0 150]  RndMeth=Simplest  InputSameDT=on
  Abs : Abs
  Gain : Gain  Gain=1/.636
  Saturation1 : Saturate  UpperLimit=Inf  LowerLimit=0
  Em_PhaAcCur : Outport
  wires:
  1-D Lookup Table/1 -> Gain/1
  Gain/1 -> Saturation1/1
  Abs/1 -> 1-D Lookup Table/1
  EM2_Trq/1 -> Abs/1
  Saturation1/1 -> Em_PhaAcCur/1

== system TM_DynamicModel_Library/DM_Emm_FlgNetSndrEna ==
  Constant : Constant  Value=0
  Emm_FlgNetSndrEna : Outport
  wires:
  Constant/1 -> Emm_FlgNetSndrEna/1

== system TM_DynamicModel_Library/DM_EngClpmp_PercPwrReq ==
  Constant : Constant  Value=0
  EngClpmp_PercPwrReq : Outport
  wires:
  Constant/1 -> EngClpmp_PercPwrReq/1

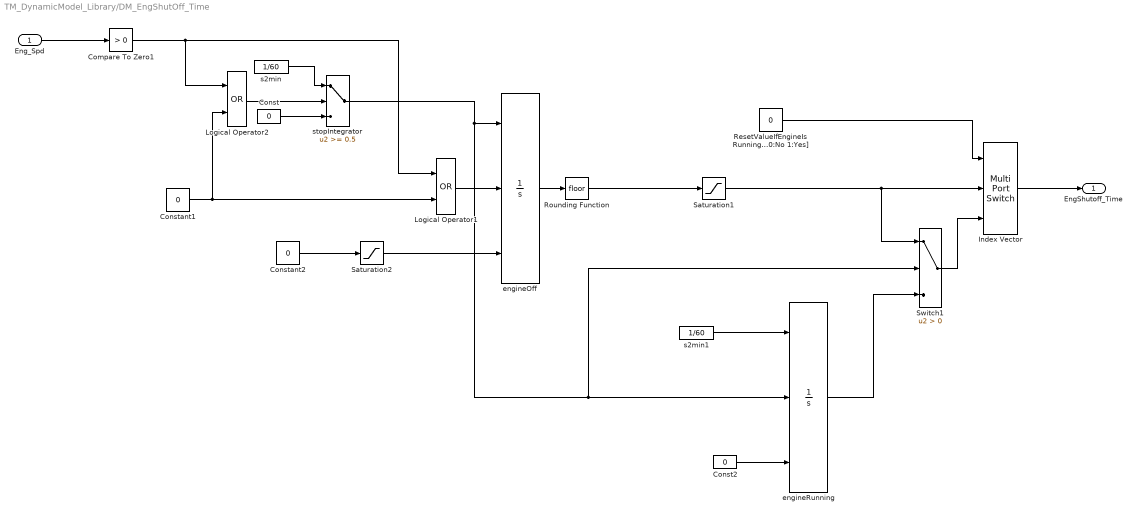
== system TM_DynamicModel_Library/DM_EngShutOff_Time ==
  Eng_Spd : Inport
  Compare To Zero1 : simulink/Logic and Bit Operations/Compare To Zero  relop=>  OutDataTypeStr=uint8
  Const : Constant  Value=0
  Const2 : Constant  Value=0
  Constant1 : Constant  Value=0
  Constant2 : Constant  Value=0
  Index Vector : MultiPortSwitch  DataPortOrder=Zero-based contiguous  Inputs=2  zeroidx=on
  Logical Operator1 : Logic  Operator=OR  AllPortsSameDT=off
  Logical Operator2 : Logic  Operator=OR  AllPortsSameDT=off
  ResetValueIfEngineIsRunning [0:No 1:Yes] : Constant  Value=0
  Rounding Function : Rounding
  Saturation1 : Saturate  UpperLimit=4095  LowerLimit=0
  Saturation2 : Saturate  UpperLimit=4095  LowerLimit=0  OutDataTypeStr=double
  Switch1 : Switch  Criteria=u2 > Threshold  SaturateOnIntegerOverflow=on
  engineOff : Integrator  ExternalReset=falling  InitialConditionSource=external
  engineRunning : Integrator  ExternalReset=falling  InitialConditionSource=external
  s2min : Constant  Value=1/60
  s2min1 : Constant  Value=1/60
  stopIntegrator : Switch  Threshold=0.5  SaturateOnIntegerOverflow=on
  EngShutoff_Time : Outport
  wires:
  Compare To Zero1/1 -> Logical Operator2/1, Logical Operator1/1
  Eng_Spd/1 -> Compare To Zero1/1
  s2min1/1 -> engineRunning/1
  Const2/1 -> engineRunning/3
  engineRunning/1 -> Switch1/3
  Switch1/1 -> Index Vector/3
  ResetValueIfEngineIsRunning [0:No 1:Yes]/1 -> Index Vector/1
  Index Vector/1 -> EngShutoff_Time/1
  Const/1 -> stopIntegrator/3
  s2min/1 -> stopIntegrator/1
  stopIntegrator/1 -> engineRunning/2, Switch1/2, engineOff/1
  Constant1/1 -> Logical Operator1/2, Logical Operator2/2
  Logical Operator1/1 -> engineOff/2
  Saturation1/1 -> Switch1/1, Index Vector/2
  engineOff/1 -> Rounding Function/1
  Rounding Function/1 -> Saturation1/1
  Logical Operator2/1 -> stopIntegrator/2
  Saturation2/1 -> engineOff/3
  Constant2/1 -> Saturation2/1

== system TM_DynamicModel_Library/DM_Eng_Actl_OpMode ==
  Eng_State_Actl : Inport
  Constant : Constant  Value=2
  Math Function : Math  Operator=pow  SaturateOnIntegerOverflow=on
  Eng_Actl_OpMode : Outport
  wires:
  Eng_State_Actl/1 -> Math Function/2
  Constant/1 -> Math Function/1
  Math Function/1 -> Eng_Actl_OpMode/1

== system TM_DynamicModel_Library/DM_Eng_Cyc_Time ==
  note: Initial condition of measurement data
  note: Sample time is 10ms
  Eng_Spd : Inport
  EIS_IgnSwState : Inport  Port=2
  Constant46 : Constant  Value=696000
  Constant47 : Constant  Value=0
  Constant48 : Constant  Value=0
  Counter_RE : Subsystem
  DM_IgnSwRun_Mode : Subsystem
  EdgeBi : Subsystem
  Eng_Run2_Mode_Sys : TM_DynamicModel_Library/DM_Eng_Run2_Mode
  Gain : Gain  Gain=0.01
  Unit Delay3 : UnitDelay  SampleTime=-1
  Eng_Cyc_Time : Outport
  wires:
  Gain/1 -> Eng_Cyc_Time/1
  Constant46/1 -> Counter_RE/3(InitVal)
  EdgeBi/1(y) -> Counter_RE/2(Reset)
  Unit Delay3/1 -> EdgeBi/2(R)
  Constant47/1 -> EdgeBi/3(IV)
  Constant48/1 -> Unit Delay3/1
  Counter_RE/1(y) -> Gain/1
  Eng_Spd/1 -> Eng_Run2_Mode_Sys/1
  Eng_Run2_Mode_Sys/1 -> Counter_RE/1(Enable)
  DM_IgnSwRun_Mode/1(IgnSwRun_Mode) -> EdgeBi/1(u)
  EIS_IgnSwState/1 -> DM_IgnSwRun_Mode/1(EIS_IgnSwState)

== system TM_DynamicModel_Library/DM_Eng_Ign_Time ==
  note: This
      | Value taken from
      | measurement
      | data
  Eng_Spd : Inport
  Eng_Trq : Inport  Port=2
  EIS_IgnSwState : Inport  Port=3
  Constant46 : Constant  Value=727300
  Constant47 : Constant  Value=0
  Constant48 : Constant  Value=0
  Counter_RE : Subsystem
  DM_AGC_ASSStop_Mode : TM_DynamicModel_Library/DM_AGC_ASSStop_Mode
  DM_Ign_Mode : Subsystem
  EdgeBi : Subsystem
  Eng_Run2_Mode_Sys : TM_DynamicModel_Library/DM_Eng_Run2_Mode
  Gain : Gain  Gain=0.01
  Logical Operator : Logic  Operator=OR  AllPortsSameDT=off  OutDataTypeStr=boolean
  Unit Delay3 : UnitDelay  SampleTime=-1
  Eng_Ign_Time : Outport
  wires:
  Constant46/1 -> Counter_RE/3(InitVal)
  EdgeBi/1(y) -> Counter_RE/2(Reset)
  Unit Delay3/1 -> EdgeBi/2(R)
  Constant47/1 -> EdgeBi/3(IV)
  Constant48/1 -> Unit Delay3/1
  Counter_RE/1(y) -> Gain/1
  Gain/1 -> Eng_Ign_Time/1
  Eng_Spd/1 -> Eng_Run2_Mode_Sys/1, DM_AGC_ASSStop_Mode/1
  Logical Operator/1 -> Counter_RE/1(Enable)
  Eng_Run2_Mode_Sys/1 -> Logical Operator/1
  DM_Ign_Mode/1(Ign_Mode) -> EdgeBi/1(u)
  EIS_IgnSwState/1 -> DM_Ign_Mode/1(EIS_IgnSwState)
  DM_AGC_ASSStop_Mode/1 -> Logical Operator/2
  Eng_Trq/1 -> DM_AGC_ASSStop_Mode/2

== system TM_DynamicModel_Library/DM_Eng_RelLoad ==
  MAF : Inport
  Eng_Spd : Inport  Port=2
  Compare To Constant : simulink/Logic and Bit Operations/Compare To Constant  relop=>=  const=400  OutDataTypeStr=uint8
  Cylinder Volume [m3] : Constant  Value=0.003
  Divide : Product  Inputs=*/
  Fixed from measurement Data : Constant  Value=62
  P/RT : Constant  Value=101325/(287*273)
  Product : Product  Inputs=3  RndMeth=Zero
  Switch : Switch  Criteria=u2 ~= 0
  kgph to kgps : Gain  Gain=1/3600
  rpm_to_cycPerSec : Gain  Gain=1/(60*2)
  toPercent : Gain  Gain=100
  Eng_RelLoad : Outport
  wires:
  Eng_Spd/1 -> rpm_to_cycPerSec/1, Compare To Constant/1
  Cylinder Volume [m3]/1 -> Product/1
  rpm_to_cycPerSec/1 -> Product/2
  P/RT/1 -> Product/3
  MAF/1 -> kgph to kgps/1
  Product/1 -> Divide/2  "TheoreticalMassFlow"
  Divide/1 -> toPercent/1
  kgph to kgps/1 -> Divide/1
  Compare To Constant/1 -> Switch/2
  toPercent/1 -> Switch/1
  Switch/1 -> Eng_RelLoad/1
  Fixed from measurement Data/1 -> Switch/3

== system TM_DynamicModel_Library/DM_Eng_RelLoad_Req ==
  MAF : Inport
  Eng_Spd : Inport  Port=2
  Compare To Constant : simulink/Logic and Bit Operations/Compare To Constant  relop=>=  const=400  OutDataTypeStr=uint8
  Cyclinder Volume [m3] : Constant  Value=0.003
  Divide : Product  Inputs=*/
  Fixed from measurement Data : Constant  Value=62
  P/RT : Constant  Value=101325/(287*273)
  Product : Product  Inputs=3  RndMeth=Zero
  Switch : Switch  Criteria=u2 ~= 0
  kgph to kgps : Gain  Gain=1/3600
  rpm_to_cycPerSec : Gain  Gain=1/(60*2)
  toPercent : Gain  Gain=100
  Eng_RelLoad_Req : Outport
  wires:
  Eng_Spd/1 -> rpm_to_cycPerSec/1, Compare To Constant/1
  Cyclinder Volume [m3]/1 -> Product/1
  rpm_to_cycPerSec/1 -> Product/2
  P/RT/1 -> Product/3
  MAF/1 -> kgph to kgps/1
  Product/1 -> Divide/2  "TheoreticalMassFlow"
  Divide/1 -> toPercent/1
  kgph to kgps/1 -> Divide/1
  Compare To Constant/1 -> Switch/2
  toPercent/1 -> Switch/1
  Switch/1 -> Eng_RelLoad_Req/1
  Fixed from measurement Data/1 -> Switch/3

== system TM_DynamicModel_Library/DM_Eng_Run2_Mode ==
  Eng_Spd : Inport
  Compare To Constant : simulink/Logic and Bit Operations/Compare To Constant  relop=>  const=300  OutDataTypeStr=uint8
  Compare To Constant1 : simulink/Logic and Bit Operations/Compare To Constant  relop=<  const=100  OutDataTypeStr=uint8
  My_SRFF : Subsystem
  Terminator : Terminator
  Eng_Run2_Mode : Outport
  wires:
  Compare To Constant1/1 -> My_SRFF/2(R)  "loc_Eng_Stop_Mode"
  Compare To Constant/1 -> My_SRFF/1(S)  "loc_Eng_Run_Mode"
  My_SRFF/2(Not_Q) -> Terminator/1
  Eng_Spd/1 -> Compare To Constant/1, Compare To Constant1/1
  My_SRFF/1(Q) -> Eng_Run2_Mode/1

== system TM_DynamicModel_Library/DM_Eng_Run_Mode ==
  Eng_Spd : Inport
  Compare To Constant : simulink/Logic and Bit Operations/Compare To Constant  relop=>=  const=40  OutDataTypeStr=uint8
  Data Type Conversion : DataTypeConversion
  Eng_Run_Mode : Outport
  wires:
  Data Type Conversion/1 -> Eng_Run_Mode/1
  Eng_Spd/1 -> Compare To Constant/1
  Compare To Constant/1 -> Data Type Conversion/1

== system TM_DynamicModel_Library/DM_Eng_Run_Time ==
  note: This value
      | set from
      | measurement data
      | for validation
      | purposes only
  Eng_Spd : Inport
  Constant46 : Constant  Value=0
  Counter_RE : Subsystem
  Eng_Run2_Mode_Sys : Subsystem
  Gain : Gain  Gain=0.01
  Logical Operator : Logic  Operator=NOT  AllPortsSameDT=off  OutDataTypeStr=boolean
  Scope : Scope  NumInputPorts=2
      settings: TimeRange=847.71  YMin=-5~-5  YMax=5~5
  Eng_Run_Time : Outport
  wires:
  Constant46/1 -> Counter_RE/3(InitVal)
  Eng_Spd/1 -> Eng_Run2_Mode_Sys/1(Eng_Spd), Scope/1  "Eng_Spd"
  Counter_RE/1(y) -> Gain/1
  Logical Operator/1 -> Counter_RE/2(Reset)
  Gain/1 -> Eng_Run_Time/1
  Eng_Run2_Mode_Sys/1(Eng_Run2_Mode) -> Counter_RE/1(Enable), Logical Operator/1, Scope/2  "Eng_Run2_mode"

== system TM_DynamicModel_Library/DM_Eng_Run_Time_ul ==
  note: This value
      | set from
      | measurement data
      | for validation
      | purposes only
  Eng_Spd : Inport
  Constant46 : Constant  Value=0
  Counter_RE : Subsystem
  Eng_Run2_Mode_Sys : TM_DynamicModel_Library/DM_Eng_Run2_Mode
  Gain : Gain  Gain=0.01
  Logical Operator : Logic  Operator=NOT  AllPortsSameDT=off  OutDataTypeStr=boolean
  Scope : Scope  NumInputPorts=2
      settings: TimeRange=847.71  YMin=-5~-5  YMax=5~5
  Eng_Run_Time_ul : Outport
  wires:
  Eng_Run2_Mode_Sys/1 -> Scope/2, Logical Operator/1, Counter_RE/1(Enable)  "Eng_Run2_mode"
  Gain/1 -> Eng_Run_Time_ul/1
  Logical Operator/1 -> Counter_RE/2(Reset)
  Counter_RE/1(y) -> Gain/1
  Eng_Spd/1 -> Scope/1, Eng_Run2_Mode_Sys/1  "Eng_Spd"
  Constant46/1 -> Counter_RE/3(InitVal)

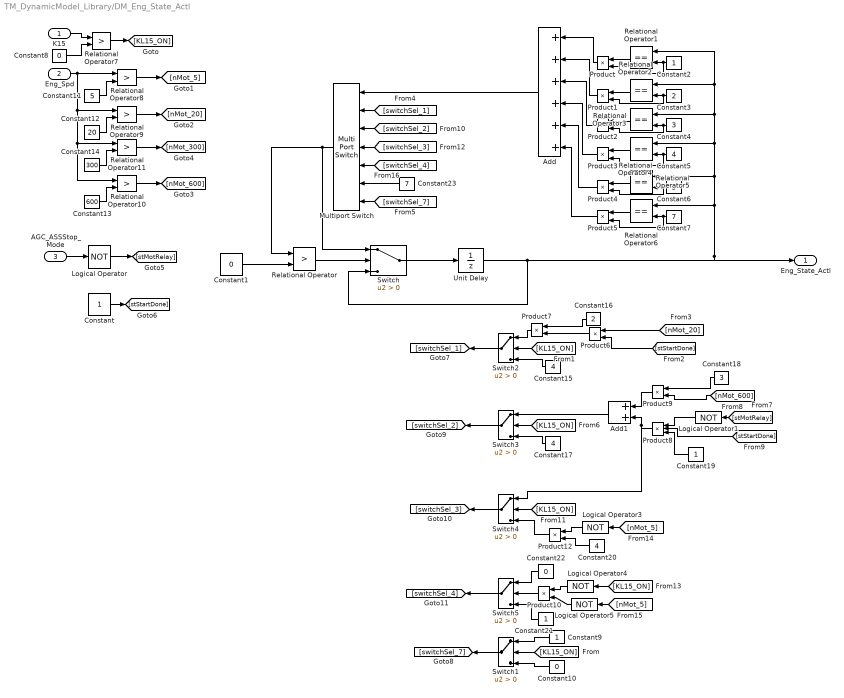
== system TM_DynamicModel_Library/DM_Eng_State_Actl ==
  K15 : Inport
  Eng_Spd : Inport  Port=2
  AGC_ASSStop_Mode : Inport  Port=3
  Add : Sum  Inputs=++++++
  Add1 : Sum
  Constant{,2,9,19,21} (5 alike) : Constant
  Constant{1,8,10,22} (4 alike) : Constant  Value=0
  Constant11 : Constant  Value=5
  Constant12 : Constant  Value=20
  Constant13 : Constant  Value=600
  Constant14 : Constant  Value=300
  Constant{5,15,17,20} (4 alike) : Constant  Value=4
  Constant16 : Constant  Value=2
  Constant18 : Constant  Value=3
  Constant23 : Constant  Value=7
  Constant3 : Constant  Value=2
  Constant4 : Constant  Value=3
  Constant6 : Constant  Value=5
  Constant7 : Constant  Value=7
  Logical Operator : Logic  Operator=NOT  AllPortsSameDT=off  OutDataTypeStr=boolean
  Logical Operator{1,3..5} (4 alike) : Logic  Operator=NOT  Inputs=1  AllPortsSameDT=off  OutDataTypeStr=boolean
  Multiport Switch : MultiPortSwitch  DataPortOrder=Specify indices  Inputs=5  DataPortIndices={1,2,3,4,5,7}  zeroidx=off
  Product{,1..7,9..10,12} (11 alike) : Product  RndMeth=Zero
  Product8 : Product  Inputs=3  RndMeth=Zero
  Relational Operator{,7..11} (6 alike) : RelationalOperator  Operator=>  OutDataTypeStr=boolean
  Relational Operator{1..6} (6 alike) : RelationalOperator  Operator===  OutDataTypeStr=boolean
  Switch{,1..5} (6 alike) : Switch  Criteria=u2 > Threshold
  Unit Delay : UnitDelay  X0=7  SampleTime=-1
  Eng_State_Actl : Outport
  wires:
  Constant1/1 -> Relational Operator/2
  Relational Operator/1 -> Switch/2
  Switch/1 -> Unit Delay/1
  Unit Delay/1 -> Switch/3, Relational Operator2/1, Relational Operator1/1, Relational Operator3/1, Relational Operator4/1, Relational Operator5/1, Relational Operator6/1, Eng_State_Actl/1
  Multiport Switch/1 -> Switch/1, Relational Operator/1
  Constant2/1 -> Relational Operator1/2, Product/2
  Constant3/1 -> Relational Operator2/2, Product1/2
  Constant4/1 -> Relational Operator3/2, Product2/2
  Constant5/1 -> Relational Operator4/2, Product3/2
  Constant6/1 -> Relational Operator5/2, Product4/2
  Constant7/1 -> Relational Operator6/2, Product5/2
  Relational Operator1/1 -> Product/1
  Relational Operator2/1 -> Product1/1
  Relational Operator3/1 -> Product2/1
  Relational Operator4/1 -> Product3/1
  Relational Operator5/1 -> Product4/1
  Relational Operator6/1 -> Product5/1
  Product/1 -> Add/1
  Product1/1 -> Add/2
  Product2/1 -> Add/3
  Product3/1 -> Add/4
  Product4/1 -> Add/5
  Product5/1 -> Add/6
  K15/1 -> Relational Operator7/1
  Constant8/1 -> Relational Operator7/2
  Relational Operator7/1 -> [KL15_ON]
  [KL15_ON] -> Switch1/2
  Eng_Spd/1 -> Relational Operator8/1, Relational Operator9/1, Relational Operator11/1, Relational Operator10/1
  Constant11/1 -> Relational Operator8/2
  Relational Operator8/1 -> [nMot_5]
  Constant12/1 -> Relational Operator9/2
  Relational Operator9/1 -> [nMot_20]
  Constant13/1 -> Relational Operator10/2
  Relational Operator10/1 -> [nMot_600]
  Constant14/1 -> Relational Operator11/2
  Relational Operator11/1 -> [nMot_300]
  Constant9/1 -> Switch1/1
  Constant10/1 -> Switch1/3
  [KL15_ON] -> Switch2/2
  Constant15/1 -> Switch2/3
  [stStartDone] -> Product6/2
  [nMot_20] -> Product6/1
  Product7/1 -> Switch2/1
  Constant16/1 -> Product7/1
  Product6/1 -> Product7/2
  Switch2/1 -> [switchSel_1]
  [switchSel_1] -> Multiport Switch/2
  Switch1/1 -> [switchSel_7]
  [switchSel_7] -> Multiport Switch/7
  Add/1 -> Multiport Switch/1
  [KL15_ON] -> Switch3/2
  Constant17/1 -> Switch3/3
  Constant18/1 -> Product9/1
  [nMot_600] -> Product9/2
  [stMotRelay] -> Logical Operator1/1
  [stStartDone] -> Product8/2
  Constant19/1 -> Product8/3
  Product9/1 -> Add1/1
  Product8/1 -> Add1/2, Switch4/1
  Add1/1 -> Switch3/1
  Switch3/1 -> [switchSel_2]
  [switchSel_2] -> Multiport Switch/3
  [KL15_ON] -> Switch4/2
  Switch4/1 -> [switchSel_3]
  [nMot_5] -> Logical Operator3/1
  Logical Operator3/1 -> Product12/1
  Constant20/1 -> Product12/2
  Product12/1 -> Switch4/3
  [switchSel_3] -> Multiport Switch/4
  Switch5/1 -> [switchSel_4]
  [KL15_ON] -> Logical Operator4/1
  [nMot_5] -> Logical Operator5/1
  Logical Operator4/1 -> Product10/1
  Logical Operator5/1 -> Product10/2
  Product10/1 -> Switch5/2
  [switchSel_4] -> Multiport Switch/5
  Constant23/1 -> Multiport Switch/6
  Logical Operator1/1 -> Product8/1
  Constant21/1 -> Switch5/3
  Constant22/1 -> Switch5/1
  Constant/1 -> [stStartDone]
  AGC_ASSStop_Mode/1 -> Logical Operator/1
  Logical Operator/1 -> [stMotRelay]
